simulink model "IceStorage_FHNW"  (R2018b)
settings: Solver=ode23  StartTime=-122*24*3600  StopTime=(365+181)*24*3600  EnableMultiTasking=on
StartFcn:
  | ticID_VsIceSTsim = tic;
StopFcn:
  | toc(ticID_VsIceSTsim)
undefined symbols (not defined in the file or in its folder): A, B, C, Davies, Dd, Hay
libraries: carnot x43, simulink x3, carsys x1
(part 2 of 2)

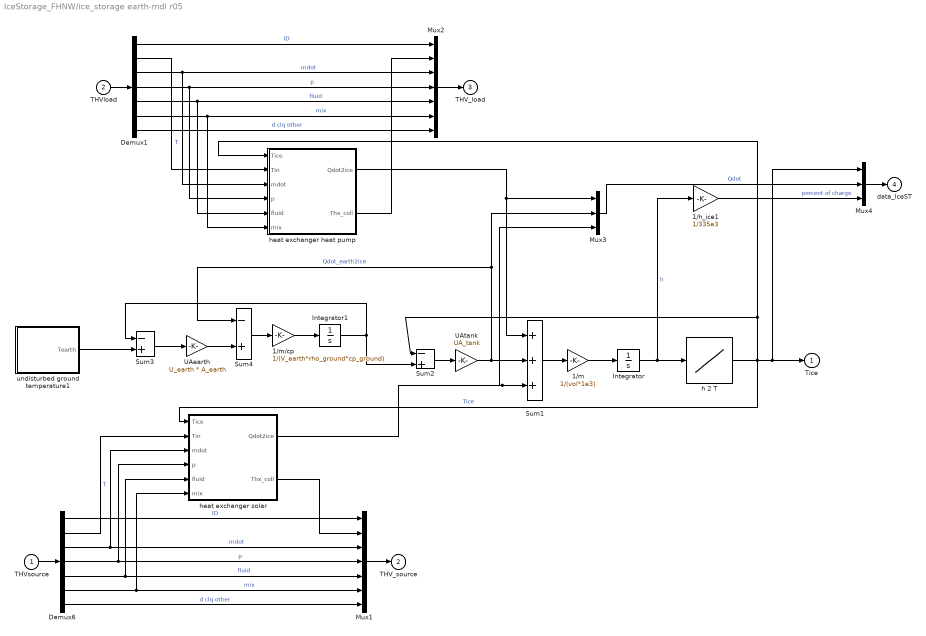
== system IceStorage_FHNW/ice_storage earth-mdl r05 ==
  THVsource : Inport
  THVload : Inport  Port=2
  1/h_ice1 : Gain  Gain=1/335e3  SaturateOnIntegerOverflow=on  OutDataTypeStr=Inherit: Same as input  ParamDataTypeStr=Inherit: Same as input
  1/m : Gain  Gain=1/(vol*1e3)  SaturateOnIntegerOverflow=on  OutDataTypeStr=Inherit: Same as input  ParamDataTypeStr=Inherit: Same as input
  1/m/cp : Gain  Gain=1/(V_earth*rho_ground*cp_ground)  SaturateOnIntegerOverflow=on  OutDataTypeStr=Inherit: Same as input  ParamDataTypeStr=Inherit: Same as input
  Demux1 : Demux  Outputs=[1 1 1 1 1 1 14]
  Demux6 : Demux  Outputs=[1 1 1 1 1 1 14]
  Integrator : Integrator  InitialCondition=h_ini
  Integrator1 : Integrator  InitialCondition=4
  Mux1 : Mux  Inputs=7
  Mux2 : Mux  Inputs=7
  Mux3 : Mux  Inputs=3
  Mux4 : Mux  Inputs=3
  Sum1 : Sum  Inputs=+++  SaturateOnIntegerOverflow=on  InputSameDT=on  OutDataTypeStr=Inherit: Same as first input
  Sum2 : Sum  Inputs=-+  SaturateOnIntegerOverflow=on  InputSameDT=on  OutDataTypeStr=Inherit: Same as first input
  Sum3 : Sum  Inputs=-+  SaturateOnIntegerOverflow=on  InputSameDT=on  OutDataTypeStr=Inherit: Same as first input
  Sum4 : Sum  Inputs=-+  SaturateOnIntegerOverflow=on  InputSameDT=on  OutDataTypeStr=Inherit: Same as first input
  UAearth : Gain  Gain=U_earth * A_earth  SaturateOnIntegerOverflow=on  OutDataTypeStr=Inherit: Same as input  ParamDataTypeStr=Inherit: Same as input
  UAtank : Gain  Gain=UA_tank  SaturateOnIntegerOverflow=on  OutDataTypeStr=Inherit: Same as input  ParamDataTypeStr=Inherit: Same as input
  h 2 T : Lookup  InputValues=[-2060*10 -2060*3 335e3 335e3+4182*10]  Table=[-10 -3 0 10]
  heat exchanger heat pump : Subsystem
  heat exchanger solar : Subsystem
  undisturbed ground temperature1 : Subsystem
  Tice : Outport  InitialOutput=0
  THV_source : Outport  Port=2  InitialOutput=0
  THV_load : Outport  Port=3  InitialOutput=0
  data_IceST : Outport  Port=4  InitialOutput=0
  wires:
  Mux3/1 -> Mux4/2  "Qdot"
  heat exchanger heat pump/1(Qdot2ice) -> Mux3/1, Sum1/1
  heat exchanger heat pump/2(Thx_coll) -> Mux2/2
  Demux1/2 -> heat exchanger heat pump/2(Tin)  "T"
  Demux1/6 -> Mux2/6, heat exchanger heat pump/6(mix)  "mix"
  Demux1/1 -> Mux2/1  "ID"
  Demux1/7 -> Mux2/7  "d clq other"
  Demux1/5 -> Mux2/5, heat exchanger heat pump/5(fluid)  "fluid"
  Demux1/4 -> Mux2/4, heat exchanger heat pump/4(p)  "p"
  Demux1/3 -> Mux2/3, heat exchanger heat pump/3(mdot)  "mdot"
  Mux2/1 -> THV_load/1
  THVload/1 -> Demux1/1
  heat exchanger solar/1(Qdot2ice) -> Mux3/3, Sum1/3
  h 2 T/1 -> Sum2/1, heat exchanger heat pump/1(Tice), heat exchanger solar/1(Tice), Mux4/1, Tice/1  "Tice"
  Integrator1/1 -> Sum3/1, Sum2/2
  1/m/cp/1 -> Integrator1/1
  Sum4/1 -> 1/m/cp/1
  UAearth/1 -> Sum4/2
  Sum3/1 -> UAearth/1
  Integrator/1 -> h 2 T/1, 1/h_ice1/1  "h"
  UAtank/1 -> Mux3/2, Sum4/1, Sum1/2  "Qdot_earth2ice"
  Sum2/1 -> UAtank/1
  Sum1/1 -> 1/m/1
  1/m/1 -> Integrator/1
  heat exchanger solar/2(Thx_coll) -> Mux1/2
  Demux6/2 -> heat exchanger solar/2(Tin)  "T"
  Demux6/6 -> heat exchanger solar/6(mix), Mux1/6  "mix"
  Demux6/1 -> Mux1/1  "ID"
  Demux6/7 -> Mux1/7  "d clq other"
  Demux6/5 -> heat exchanger solar/5(fluid), Mux1/5  "fluid"
  Demux6/4 -> heat exchanger solar/4(p), Mux1/4  "p"
  Demux6/3 -> heat exchanger solar/3(mdot), Mux1/3  "mdot"
  Mux1/1 -> THV_source/1
  THVsource/1 -> Demux6/1
  Mux4/1 -> data_IceST/1
  1/h_ice1/1 -> Mux4/3  "percent of charge"
  undisturbed ground temperature1/1(Tearth) -> Sum3/2

== system IceStorage_FHNW/measure_T ==
  THV_in : Inport
  heat capacity : StateSpace  A=-tc  B=tc  D=0  InitialCondition=t0
  select temperature : Selector  InputPortWidth=20  IndexOptions=Index vector (dialog)  Indices=[2]  OutputSizes=1
  T : Outport  InitialOutput=0
  wires:
  THV_in/1 -> select temperature/1
  select temperature/1 -> heat capacity/1
  heat capacity/1 -> T/1

== system IceStorage_FHNW/measure_T1 ==
  THV_in : Inport
  heat capacity : StateSpace  A=-tc  B=tc  D=0  InitialCondition=t0
  select temperature : Selector  InputPortWidth=20  IndexOptions=Index vector (dialog)  Indices=[2]  OutputSizes=1
  T : Outport  InitialOutput=0
  wires:
  heat capacity/1 -> T/1
  select temperature/1 -> heat capacity/1
  THV_in/1 -> select temperature/1

== system IceStorage_FHNW/measure_T2 ==
  THV_in : Inport
  heat capacity : StateSpace  A=-tc  B=tc  D=0  InitialCondition=t0
  select temperature : Selector  InputPortWidth=20  IndexOptions=Index vector (dialog)  Indices=[2]  OutputSizes=1
  T : Outport  InitialOutput=0
  wires:
  THV_in/1 -> select temperature/1
  select temperature/1 -> heat capacity/1
  heat capacity/1 -> T/1

== system IceStorage_FHNW/measure_T3 ==
  THV_in : Inport
  heat capacity : StateSpace  A=-tc  B=tc  D=0  InitialCondition=t0
  select temperature : Selector  InputPortWidth=20  IndexOptions=Index vector (dialog)  Indices=[2]  OutputSizes=1
  T : Outport  InitialOutput=0
  wires:
  THV_in/1 -> select temperature/1
  select temperature/1 -> heat capacity/1
  heat capacity/1 -> T/1

== system IceStorage_FHNW/measure_T4 ==
  THV_in : Inport
  heat capacity : StateSpace  A=-tc  B=tc  D=0  InitialCondition=t0
  select temperature : Selector  InputPortWidth=20  IndexOptions=Index vector (dialog)  Indices=[2]  OutputSizes=1
  T : Outport  InitialOutput=0
  wires:
  THV_in/1 -> select temperature/1
  select temperature/1 -> heat capacity/1
  heat capacity/1 -> T/1

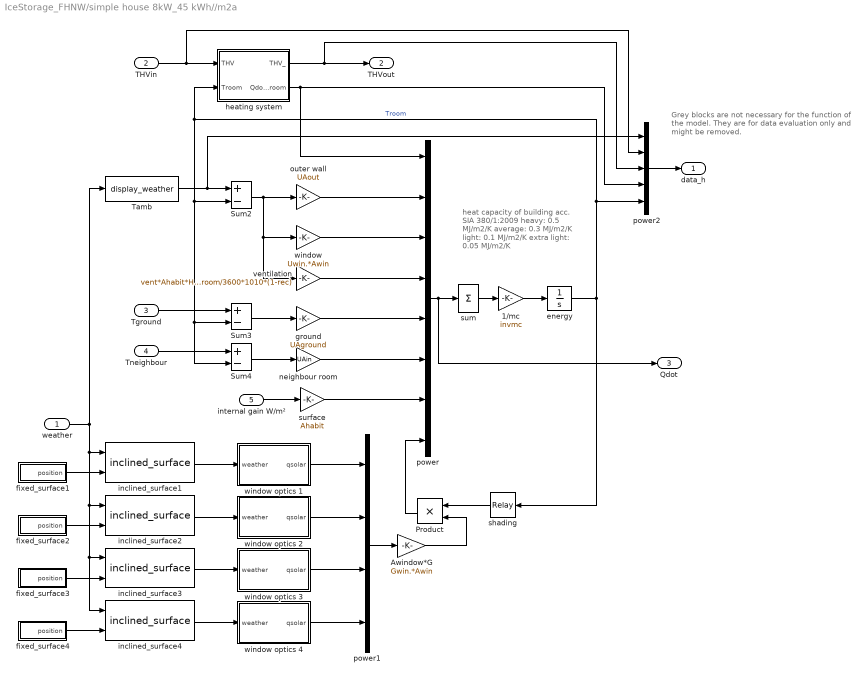
== system IceStorage_FHNW/simple house 8kW_45 kWh//m2a ==
  note: Grey blocks are not necessary for the function
      | of the model. They are for data evaluation only
      | and might be removed.
  note: heat capacity of building
      | acc. SIA 380/1:2009
      | heavy:          0.5 MJ/m2/K
      | average:       0.3 MJ/m2/K
      | light:            0.1 MJ/m2/K
      | extra light:  0.05 MJ/m2/K
  weather : Inport
  THVin : Inport  Port=2
  Tground : Inport  Port=3
  Tneighbour : Inport  Port=4
  internal gain W/m² : Inport  Port=5
  1/mc : Gain  Gain=invmc  SaturateOnIntegerOverflow=on  OutDataTypeStr=Inherit: Same as input  ParamDataTypeStr=Inherit: Same as input
  Awindow*G : Gain  Gain=Gwin.*Awin  SaturateOnIntegerOverflow=on  OutDataTypeStr=Inherit: Same as input  ParamDataTypeStr=Inherit: Same as input
  Product : Product  RndMeth=Zero
  Sum2 : Sum  Inputs=+-  SaturateOnIntegerOverflow=on  InputSameDT=on  OutDataTypeStr=Inherit: Same as first input
  Sum3 : Sum  Inputs=+-  SaturateOnIntegerOverflow=on  InputSameDT=on  OutDataTypeStr=Inherit: Same as first input
  Sum4 : Sum  Inputs=+-  SaturateOnIntegerOverflow=on  InputSameDT=on  OutDataTypeStr=Inherit: Same as first input
  Tamb : carnot/outputs/display_weather  pos=off  sun_dir=off  sun_dfu=off  rad=off  ta=on  ts=off  pre=off  rh=off  ci=off  p=off  ws=off  wd=off  col=off
      settings: SourceProductName=Carnot
  energy : Integrator  InitialCondition=tini
  fixed_surface1 : Subsystem  mask(fixed surface){colangle=90, colazi=AziWin(1), colrot=0}
      mask prompts: colangle "collector slope (0° = horizontal) [degree]"; colazi "collector azimuth (0° = south, -90° = east) [degree]"; colrot "collector rotation angle [degree]"
      mask help:
      | Set collector or surface to a fixed position.
      | All angles in degrees.
      mask init:
      | colangle = min(180, max(-180, colangle));
      | colazi = min(180, max(-180, colazi));
      | colrot = min(180, max(-180, colrot));
      mask Help: eval('htmlhelp (''chap_4_2f.htm#fixed_surface'')')
  fixed_surface2 : Subsystem  mask(fixed surface){colangle=90, colazi=AziWin(2), colrot=0}
      mask prompts: colangle "collector slope (0° = horizontal) [degree]"; colazi "collector azimuth (0° = south, -90° = east) [degree]"; colrot "collector rotation angle [degree]"
      mask help:
      | Set collector or surface to a fixed position.
      | All angles in degrees.
      mask init:
      | colangle = min(180, max(-180, colangle));
      | colazi = min(180, max(-180, colazi));
      | colrot = min(180, max(-180, colrot));
      mask Help: eval('htmlhelp (''chap_4_2f.htm#fixed_surface'')')
  fixed_surface3 : Subsystem  mask(fixed surface){colangle=90, colazi=AziWin(3), colrot=0}
      mask prompts: colangle "collector slope (0° = horizontal) [degree]"; colazi "collector azimuth (0° = south, -90° = east) [degree]"; colrot "collector rotation angle [degree]"
      mask help:
      | Set collector or surface to a fixed position.
      | All angles in degrees.
      mask init:
      | colangle = min(180, max(-180, colangle));
      | colazi = min(180, max(-180, colazi));
      | colrot = min(180, max(-180, colrot));
      mask Help: eval('htmlhelp (''chap_4_2f.htm#fixed_surface'')')
  fixed_surface4 : Subsystem  mask(fixed surface){colangle=90, colazi=AziWin(4), colrot=0}
      mask prompts: colangle "collector slope (0° = horizontal) [degree]"; colazi "collector azimuth (0° = south, -90° = east) [degree]"; colrot "collector rotation angle [degree]"
      mask help:
      | Set collector or surface to a fixed position.
      | All angles in degrees.
      mask init:
      | colangle = min(180, max(-180, colangle));
      | colazi = min(180, max(-180, colazi));
      | colrot = min(180, max(-180, colrot));
      mask Help: eval('htmlhelp (''chap_4_2f.htm#fixed_surface'')')
  ground : Gain  Gain=UAground  SaturateOnIntegerOverflow=on  OutDataTypeStr=Inherit: Same as input  ParamDataTypeStr=Inherit: Same as input
  heating system : Subsystem
  inclined_surface{1..4} (4 alike) : carnot/weather/inclined_surface  sky=Hay-Davies  reflect=0.2
      settings: SourceProductName=Carnot
  neighbour room : Gain  Gain=UAin  SaturateOnIntegerOverflow=on  OutDataTypeStr=Inherit: Same as input  ParamDataTypeStr=Inherit: Same as input
  outer wall : Gain  Gain=UAout  SaturateOnIntegerOverflow=on  OutDataTypeStr=Inherit: Same as input  ParamDataTypeStr=Inherit: Same as input
  power : Mux  Inputs=8
  power1 : Mux
  power2 : Mux  Inputs=5
  shading : Relay  OnSwitchValue=tini+4  OffSwitchValue=tini+3.5  OnOutputValue=1-shade  OffOutputValue=1
  sum : Sum  Inputs=1  SaturateOnIntegerOverflow=on  InputSameDT=on  OutDataTypeStr=Inherit: Same as first input
  surface : Gain  Gain=Ahabit  SaturateOnIntegerOverflow=on  OutDataTypeStr=Inherit: Same as input  ParamDataTypeStr=Inherit: Same as input
  ventilation : Gain  Gain=vent*Ahabit*Hroom/3600*1010*(1-rec)  SaturateOnIntegerOverflow=on  OutDataTypeStr=Inherit: Same as input  ParamDataTypeStr=Inherit: Same as input
  window : Gain  Gain=Uwin.*Awin  SaturateOnIntegerOverflow=on  OutDataTypeStr=Inherit: Same as input  ParamDataTypeStr=Inherit: Same as input
  window optics 1 : Subsystem
  window optics 2 : Subsystem
  window optics 3 : Subsystem
  window optics 4 : Subsystem
  data_h : Outport  InitialOutput=0
  THVout : Outport  Port=2  InitialOutput=0
  Qdot : Outport  Port=3  InitialOutput=0
  wires:
  1/mc/1 -> energy/1
  energy/1 -> Sum4/2, Sum3/2, Sum2/2, heating system/2(Troom), power2/5, shading/1  "Troom"
  sum/1 -> 1/mc/1
  inclined_surface4/1 -> window optics 4/1(weather)
  fixed_surface4/1(position) -> inclined_surface4/2
  inclined_surface3/1 -> window optics 3/1(weather)
  fixed_surface3/1(position) -> inclined_surface3/2
  inclined_surface2/1 -> window optics 2/1(weather)
  fixed_surface2/1(position) -> inclined_surface2/2
  power1/1 -> Awindow*G/1
  inclined_surface1/1 -> window optics 1/1(weather)
  fixed_surface1/1(position) -> inclined_surface1/2
  surface/1 -> power/7
  internal gain W/m²/1 -> surface/1
  neighbour room/1 -> power/6
  ground/1 -> power/5
  ventilation/1 -> power/4
  window/1 -> power/3
  Tneighbour/1 -> Sum4/1
  Sum4/1 -> neighbour room/1
  Tground/1 -> Sum3/1
  Sum3/1 -> ground/1
  heating system/1(THV_) -> THVout/1, power2/3
  THVin/1 -> heating system/1(THV), power2/2
  heating system/2(Qdot2room) -> power/1, power2/4
  power/1 -> sum/1, Qdot/1
  weather/1 -> inclined_surface4/1, inclined_surface3/1, inclined_surface2/1, inclined_surface1/1, Tamb/1
  Tamb/1 -> Sum2/1, power2/1
  outer wall/1 -> power/2
  Sum2/1 -> ventilation/1, window/1, outer wall/1
  power2/1 -> data_h/1
  shading/1 -> Product/1
  Awindow*G/1 -> Product/2
  Product/1 -> power/8
  window optics 1/1(qsolar) -> power1/1
  window optics 2/1(qsolar) -> power1/2
  window optics 3/1(qsolar) -> power1/3
  window optics 4/1(qsolar) -> power1/4

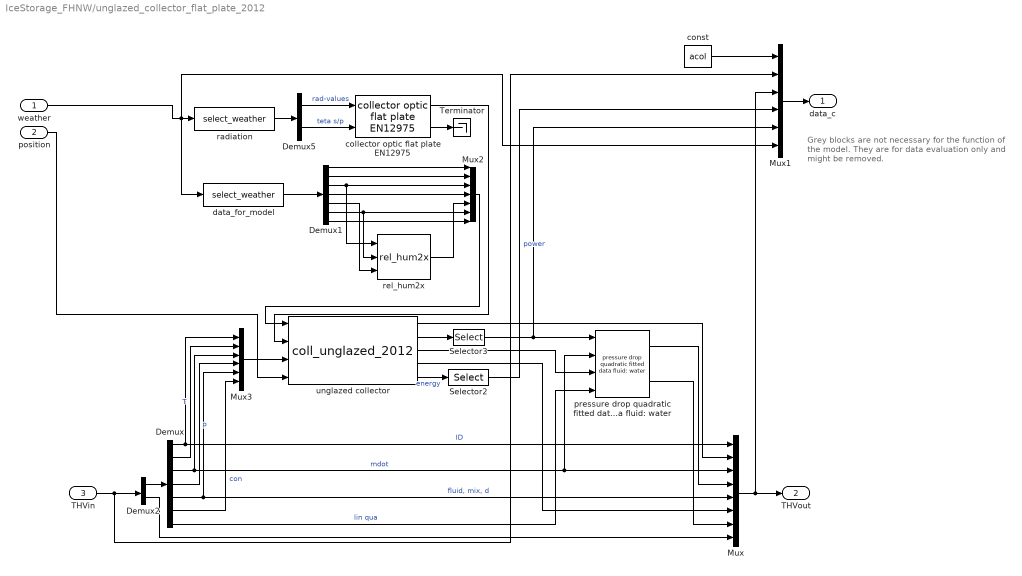
== system IceStorage_FHNW/unglazed_collector_flat_plate_2012 ==
  note: Grey blocks are not necessary for the function
      | of the model. They are for data evaluation only
      | and might be removed.
  weather : Inport
  position : Inport  Port=2
  THVin : Inport  Port=3
  Demux : Demux  Outputs=[1 1 1 1 3 1 2]
  Demux1 : Demux  Outputs=7
  Demux2 : Demux  Outputs=[10 10]
  Demux5 : Demux  Outputs=[5 2]
  Mux : Mux  Inputs=8
  Mux1 : Mux  Inputs=[1 20 20 1 1 -1]
  Mux2 : Mux  Inputs=7
  Mux3 : Mux  Inputs=6
  Selector2 : Selector  InputPortWidth=4  IndexOptions=Index vector (dialog)  Indices=[3]  OutputSizes=1
  Selector3 : Selector  InputPortWidth=6  IndexOptions=Index vector (dialog)  Indices=[6]  OutputSizes=1
  Terminator : Terminator
  collector optic flat plate EN12975 : carnot/heat_source/incidence angle modifier (IAM)/collector optic flat plate EN12975  b0=0  Kd=1
      settings: SourceProductName=Carnot
  const : Constant  Value=acol
  data_for_model : carnot/weather/select_weather  v=[16 17 5:7 10 11]  type_index=index of weather data vectors for CARNOT versions >= 5.1
      settings: SourceProductName=Carnot
  pressure drop quadratic fitted data fluid: water : carnot/heat_source/pressure drop of collector/pressure drop quadratic fitted data fluid: water  b=0.006201*3.6e5  a=0.000096*1.296e9  aonecol=2  acol=acol
      settings: SourceProductName=Carnot
  radiation : carnot/weather/select_weather  v=[1 2 13 16 17 14 15]  type_index=index of weather data vectors for CARNOT versions >= 5.1
      settings: SourceProductName=Carnot
  rel_hum2x : carnot/basics/rel_hum2x
      settings: SourceProductName=Carnot
  unglazed collector : S-Function  FunctionName=coll_unglazed_2012  Parameters=acol, uc0, uc1, uc0loss, uc1loss, uc0gain, uc1gain, e_sky, uc1eta0, hi, c_abs, c_fl, length, tini, nodes  SFunctionDeploymentMode=off  EnableBusSupport=off
  data_c : Outport  InitialOutput=0
  THVout : Outport  Port=2  InitialOutput=0
  wires:
  collector optic flat plate EN12975/1 -> unglazed collector/2
  Mux2/1 -> unglazed collector/1
  Demux1/4 -> Mux2/4
  rel_hum2x/1 -> Mux2/5
  Demux1/7 -> Mux2/7
  Demux1/2 -> Mux2/2
  Demux1/1 -> Mux2/1
  Demux1/5 -> rel_hum2x/3
  Demux1/6 -> Mux2/6, rel_hum2x/2
  Demux1/3 -> Mux2/3, rel_hum2x/1
  data_for_model/1 -> Demux1/1
  collector optic flat plate EN12975/2 -> Terminator/1
  unglazed collector/1 -> Mux/2
  unglazed collector/2 -> Selector3/1
  unglazed collector/3 -> pressure drop quadratic fitted data fluid: water/3
  unglazed collector/4 -> Mux/6
  Mux/1 -> THVout/1, Mux1/3
  Demux/3 -> Mux3/3, Mux/3, pressure drop quadratic fitted data fluid: water/2  "mdot"
  Demux/7 -> pressure drop quadratic fitted data fluid: water/4  "lin qua"
  Mux3/1 -> unglazed collector/3
  Demux5/2 -> collector optic flat plate EN12975/2  "teta s/p"
  Demux5/1 -> collector optic flat plate EN12975/1  "rad-values"
  radiation/1 -> Demux5/1
  position/1 -> unglazed collector/4
  weather/1 -> Mux1/6, radiation/1, data_for_model/1
  Demux/5 -> Mux/5, Mux3/5  "fluid, mix, d"
  Demux/1 -> Mux3/1, Mux/1  "ID"
  Demux2/1 -> Demux/1
  THVin/1 -> Demux2/1, Mux1/2
  Demux/4 -> Mux3/4  "p"
  Demux/2 -> Mux3/2  "T"
  Demux/6 -> Mux3/6  "con"
  pressure drop quadratic fitted data fluid: water/1 -> Mux/4
  Demux2/2 -> Mux/8
  pressure drop quadratic fitted data fluid: water/2 -> Mux/7
  unglazed collector/5 -> Selector2/1  "energy"
  Selector2/1 -> Mux1/4  "power"
  const/1 -> Mux1/1
  Mux1/1 -> data_c/1
  Selector3/1 -> pressure drop quadratic fitted data fluid: water/1, Mux1/5

== system IceStorage_FHNW/Viessmann_CVW_DHW_390_Liter/multiport storage ==
  Tamb : Inport
  port1 : Inport  Port=2
  port2 : Inport  Port=3
  port3 : Inport  Port=4
  S-Function : S-Function  FunctionName=generic_store  Parameters="d(1), d(2), 0, 0, pos, u(1), u(2), u(3), axialcond,  tinitial,  nodes, nport, 0, sensors"  SFunctionDeploymentMode=off  EnableBusSupport=off
  Tnodes : Outport  InitialOutput=0
  Energy : Outport  Port=2  InitialOutput=0
  "[T p]1" : Outport  Port=3  InitialOutput=0
  "[T p]2" : Outport  Port=4  InitialOutput=0
  "[T p]3" : Outport  Port=5  InitialOutput=0
  wires:
  S-Function/1 -> Tnodes/1
  port2/1 -> S-Function/3
  port1/1 -> S-Function/2
  Tamb/1 -> S-Function/1
  port3/1 -> S-Function/4
  S-Function/3 -> "[T p]1"/1
  S-Function/4 -> "[T p]2"/1
  S-Function/5 -> "[T p]3"/1
  S-Function/2 -> Energy/1

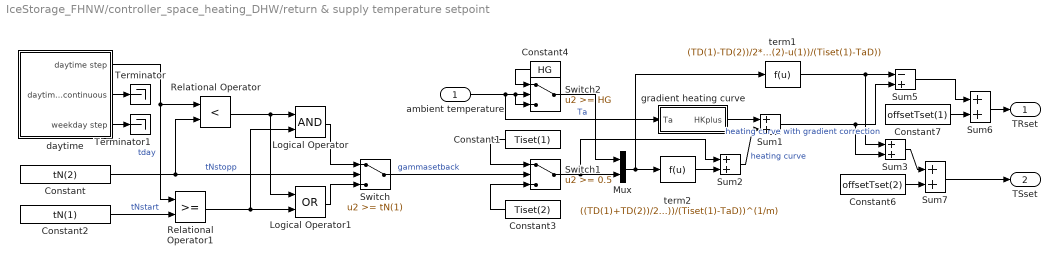
== system IceStorage_FHNW/controller_space_heating_DHW/return & supply temperature setpoint ==
  ambient temperature : Inport
  Constant : Constant  Value=tN(2)
  Constant1 : Constant  Value=Tiset(1)
  Constant2 : Constant  Value=tN(1)
  Constant3 : Constant  Value=Tiset(2)
  Constant4 : Constant  Value=HG
  Constant6 : Constant  Value=offsetTset(2)
  Constant7 : Constant  Value=offsetTset(1)
  Logical Operator : Logic
  Logical Operator1 : Logic  Operator=OR
  Mux : Mux  Inputs=2
  Relational Operator : RelationalOperator  Operator=<  RndMeth=Nearest  InputSameDT=on
  Relational Operator1 : RelationalOperator  RndMeth=Nearest  InputSameDT=on
  Sum{1..3,6..7} (5 alike) : Sum  SaturateOnIntegerOverflow=on  InputSameDT=on  OutDataTypeStr=Inherit: Same as first input
  Sum5 : Sum  Inputs=-+  SaturateOnIntegerOverflow=on  InputSameDT=on  OutDataTypeStr=Inherit: Same as first input
  Switch : Switch  Threshold=tN(1)  SaturateOnIntegerOverflow=on  InputSameDT=on
  Switch1 : Switch  Threshold=0.5  SaturateOnIntegerOverflow=on  InputSameDT=on
  Switch2 : Switch  Threshold=HG  SaturateOnIntegerOverflow=on  InputSameDT=on
  Terminator : Terminator
  Terminator1 : Terminator
  daytime : Subsystem
      mask help:
      | Evaluates the daytime and the weekday out of the simulation time.
      | The Decimation of the clock has to be adjusted under the mask in the clock parameter menu.
      | Output in seconds [s]
      mask Help:
      | created        10.2001  FHBB - IfE, suw
      | updated  22.01.2002  FHBB - IfE, suw / daytime continuous
      |                                                              / weekday step
      | 
      | The first weekday with simulation starttime zero is monday.
  gradient heating curve : Subsystem
  term1 : Fcn  Expr=(TD(1)-TD(2))/2*((u(2)-u(1))/(Tiset(1)-TaD))
  term2 : Fcn  Expr=((TD(1)+TD(2))/2-Tiset(1))*((u(2)-u(1))/(Tiset(1)-TaD))^(1/m)
  TRset : Outport
  TSset : Outport  Port=2
  wires:
  Switch2/1 -> Mux/1
  Constant4/1 -> Switch2/1
  Constant7/1 -> Sum6/2
  Constant6/1 -> Sum7/2
  Sum6/1 -> TRset/1
  Sum7/1 -> TSset/1
  term1/1 -> Sum5/1, Sum3/1
  Sum2/1 -> Sum1/2  "heating curve"
  Switch/1 -> Switch1/2  "gammasetback"
  Logical Operator1/1 -> Switch/3
  Switch1/1 -> Mux/2, Sum2/1
  Constant3/1 -> Switch1/3
  Constant1/1 -> Switch1/1
  Logical Operator/1 -> Switch/1
  Relational Operator1/1 -> Logical Operator1/2, Logical Operator/2
  Relational Operator/1 -> Logical Operator/1, Logical Operator1/1
  Constant2/1 -> Relational Operator1/2  "tNstart"
  Constant/1 -> Relational Operator/2, Switch/2  "tNstopp"
  daytime/1(daytime step) -> Relational Operator/1, Relational Operator1/1  "tday"
  ambient temperature/1 -> Switch2/2, Switch2/3, gradient heating curve/1(Ta)  "Ta"
  Mux/1 -> term2/1, term1/1
  term2/1 -> Sum2/2
  daytime/2(daytime continuous) -> Terminator/1
  daytime/3(weekday step) -> Terminator1/1
  Sum5/1 -> Sum6/1
  Sum3/1 -> Sum7/1
  Sum1/1 -> Sum5/2, Sum3/2  "heating curve with gradient correction"
  gradient heating curve/1(HKplus) -> Sum1/1

== system IceStorage_FHNW/controller_space_heating_DHW/schedule modi ==
  Clock : Clock
  Constant : Constant  Value=sim_start_time
  Fcn1 : Fcn  Expr=rem(u[1],period)
  Look-Up Table1 : Lookup  InputValues=rep_seq_t - min(rep_seq_t)  Table=rep_seq_y  SaturateOnIntegerOverflow=on
  Sum : Sum  Inputs=+-  SaturateOnIntegerOverflow=on  InputSameDT=on  OutDataTypeStr=Inherit: Same as first input
  Out1 : Outport
  wires:
  Fcn1/1 -> Look-Up Table1/1
  Look-Up Table1/1 -> Out1/1
  Sum/1 -> Fcn1/1
  Clock/1 -> Sum/1
  Constant/1 -> Sum/2

== system IceStorage_FHNW/controller_space_heating_DHW/value balance & hysteresis ==
  T : Inport
  Tset : Inport  Port=2
  Data Type Conversion3 : DataTypeConversion  OutDataTypeStr=double
  MinMax : MinMax  Function=max  Inputs=2  SaturateOnIntegerOverflow=on  InputSameDT=on
  Product : Product  SaturateOnIntegerOverflow=on  RndMeth=Zero  InputSameDT=on  OutDataTypeStr=Inherit: Same as first input
  Relational Operator2 : RelationalOperator  Operator=<=  RndMeth=Nearest  InputSameDT=on
  Relay : Relay  OnSwitchValue=deltaTRset(1)  OffSwitchValue=deltaTRset(2)
  Sum1 : Sum  Inputs=-+  SaturateOnIntegerOverflow=on  InputSameDT=on  OutDataTypeStr=Inherit: Same as first input
  Tmax option : Constant  Value=200
  signal : Outport
  wires:
  Data Type Conversion3/1 -> Product/2
  Sum1/1 -> Relay/1
  Tmax option/1 -> Relational Operator2/2
  MinMax/1 -> Relational Operator2/1
  Relay/1 -> Product/1  "gammaRset"
  Relational Operator2/1 -> Data Type Conversion3/1
  T/1 -> MinMax/1, Sum1/1  "T"
  Product/1 -> signal/1
  Tset/1 -> MinMax/2, Sum1/2  "Tset"

== system IceStorage_FHNW/controller_space_heating_DHW/value balance & hysteresis1 ==
  T : Inport
  Tset : Inport  Port=2
  Data Type Conversion3 : DataTypeConversion  OutDataTypeStr=double
  MinMax : MinMax  Function=max  Inputs=2  SaturateOnIntegerOverflow=on  InputSameDT=on
  Product : Product  SaturateOnIntegerOverflow=on  RndMeth=Zero  InputSameDT=on  OutDataTypeStr=Inherit: Same as first input
  Relational Operator2 : RelationalOperator  Operator=<=  RndMeth=Nearest  InputSameDT=on
  Relay : Relay  OnSwitchValue=deltaTRset(1)  OffSwitchValue=deltaTRset(2)
  Sum1 : Sum  Inputs=-+  SaturateOnIntegerOverflow=on  InputSameDT=on  OutDataTypeStr=Inherit: Same as first input
  Tmax option : Constant  Value=200
  signal : Outport
  wires:
  Data Type Conversion3/1 -> Product/2
  Tset/1 -> Sum1/2, MinMax/2  "Tset"
  Product/1 -> signal/1
  T/1 -> Sum1/1, MinMax/1  "T"
  Relational Operator2/1 -> Data Type Conversion3/1
  Relay/1 -> Product/1  "gammaRset"
  MinMax/1 -> Relational Operator2/1
  Tmax option/1 -> Relational Operator2/2
  Sum1/1 -> Relay/1

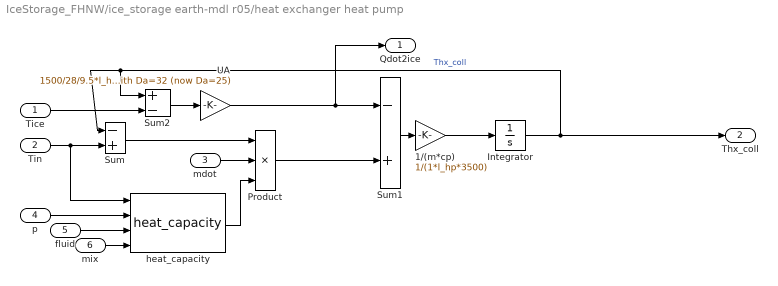
== system IceStorage_FHNW/ice_storage earth-mdl r05/heat exchanger heat pump ==
  Tice : Inport
  Tin : Inport  Port=2
  mdot : Inport  Port=3
  p : Inport  Port=4
  fluid : Inport  Port=5
  mix : Inport  Port=6
  1/(m*cp) : Gain  Gain=1/(1*l_hp*3500)  SaturateOnIntegerOverflow=on  OutDataTypeStr=Inherit: Same as input  ParamDataTypeStr=Inherit: Same as input
  Integrator : Integrator
  Product : Product  Inputs=3  SaturateOnIntegerOverflow=on  InputSameDT=on  OutDataTypeStr=Inherit: Same as first input
  Sum : Sum  Inputs=-+  SaturateOnIntegerOverflow=on  InputSameDT=on  OutDataTypeStr=Inherit: Same as first input
  Sum1 : Sum  Inputs=-+  SaturateOnIntegerOverflow=on  InputSameDT=on  OutDataTypeStr=Inherit: Same as first input
  Sum2 : Sum  Inputs=+-  SaturateOnIntegerOverflow=on  InputSameDT=on  OutDataTypeStr=Inherit: Same as first input
  UA : Gain  Gain="1500/28/9.5*l_hp*25/32            % 1.5 kW at 9 K on a 28 m tube with Da=32 (now Da=25)"  SaturateOnIntegerOverflow=on  OutDataTypeStr=Inherit: Same as input  ParamDataTypeStr=Inherit: Same as input
  heat_capacity : carnot/loads/simple house/heating system/radiator/heat_capacity
      settings: SourceProductName=Carnot
  Qdot2ice : Outport
  Thx_coll : Outport  Port=2
  wires:
  Tin/1 -> Sum/2, heat_capacity/1
  Integrator/1 -> Sum/1, Sum2/1, Thx_coll/1  "Thx_coll"
  Sum1/1 -> 1/(m*cp)/1
  Product/1 -> Sum1/2
  heat_capacity/1 -> Product/3
  Sum/1 -> Product/1
  Sum2/1 -> UA/1
  mdot/1 -> Product/2
  p/1 -> heat_capacity/2
  fluid/1 -> heat_capacity/3
  mix/1 -> heat_capacity/4
  Tice/1 -> Sum2/2
  1/(m*cp)/1 -> Integrator/1
  UA/1 -> Sum1/1, Qdot2ice/1

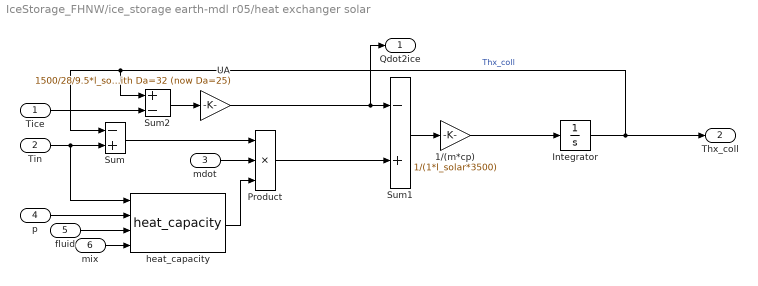
== system IceStorage_FHNW/ice_storage earth-mdl r05/heat exchanger solar ==
  Tice : Inport
  Tin : Inport  Port=2
  mdot : Inport  Port=3
  p : Inport  Port=4
  fluid : Inport  Port=5
  mix : Inport  Port=6
  1/(m*cp) : Gain  Gain=1/(1*l_solar*3500)  SaturateOnIntegerOverflow=on  OutDataTypeStr=Inherit: Same as input  ParamDataTypeStr=Inherit: Same as input
  Integrator : Integrator
  Product : Product  Inputs=3  SaturateOnIntegerOverflow=on  InputSameDT=on  OutDataTypeStr=Inherit: Same as first input
  Sum : Sum  Inputs=-+  SaturateOnIntegerOverflow=on  InputSameDT=on  OutDataTypeStr=Inherit: Same as first input
  Sum1 : Sum  Inputs=-+  SaturateOnIntegerOverflow=on  InputSameDT=on  OutDataTypeStr=Inherit: Same as first input
  Sum2 : Sum  Inputs=+-  SaturateOnIntegerOverflow=on  InputSameDT=on  OutDataTypeStr=Inherit: Same as first input
  UA : Gain  Gain="1500/28/9.5*l_solar*25/32            % 1.5 kW at 9 K on a 28 m tube with Da=32 (now Da=25)"  SaturateOnIntegerOverflow=on  OutDataTypeStr=Inherit: Same as input  ParamDataTypeStr=Inherit: Same as input
  heat_capacity : carnot/loads/simple house/heating system/radiator/heat_capacity
      settings: SourceProductName=Carnot
  Qdot2ice : Outport
  Thx_coll : Outport  Port=2
  wires:
  Tice/1 -> Sum2/2
  mix/1 -> heat_capacity/4
  fluid/1 -> heat_capacity/3
  p/1 -> heat_capacity/2
  mdot/1 -> Product/2
  Sum2/1 -> UA/1
  Sum/1 -> Product/1
  heat_capacity/1 -> Product/3
  Product/1 -> Sum1/2
  Sum1/1 -> 1/(m*cp)/1
  Integrator/1 -> Thx_coll/1, Sum2/1, Sum/1  "Thx_coll"
  Tin/1 -> heat_capacity/1, Sum/2
  1/(m*cp)/1 -> Integrator/1
  UA/1 -> Qdot2ice/1, Sum1/1

== system IceStorage_FHNW/ice_storage earth-mdl r05/undisturbed ground temperature1 ==
  Fcn : Fcn  Expr=u(1) - u(2)*exp(-u(3)/u(4))*cos(2*pi*(u(5)-u(6)*3600)/(365*24*3600) - u(3)/u(4)) + 0.03*u(3)
  Mux : Mux  Inputs=6
  Tmeanoutside : Constant  Value=Tmeanoutside
  delta_grd : Constant  Value=delta_grd
  deltathetae : Constant  Value=deltathetae
  depth of center of wall : Constant  Value=ztilde
  time : Clock
  tshift : Constant  Value=tshift
  Tearth : Outport
  wires:
  Fcn/1 -> Tearth/1
  Mux/1 -> Fcn/1
  tshift/1 -> Mux/6
  time/1 -> Mux/5
  delta_grd/1 -> Mux/4
  depth of center of wall/1 -> Mux/3
  deltathetae/1 -> Mux/2
  Tmeanoutside/1 -> Mux/1

== system IceStorage_FHNW/simple house 8kW_45 kWh//m2a/fixed_surface1 ==
  collector position : Constant  Value=[colangle colazi colrot]
  position : Outport  InitialOutput=0
  wires:
  collector position/1 -> position/1

== system IceStorage_FHNW/simple house 8kW_45 kWh//m2a/fixed_surface2 ==
  collector position : Constant  Value=[colangle colazi colrot]
  position : Outport  InitialOutput=0
  wires:
  collector position/1 -> position/1

== system IceStorage_FHNW/simple house 8kW_45 kWh//m2a/fixed_surface3 ==
  collector position : Constant  Value=[colangle colazi colrot]
  position : Outport  InitialOutput=0
  wires:
  collector position/1 -> position/1

== system IceStorage_FHNW/simple house 8kW_45 kWh//m2a/fixed_surface4 ==
  collector position : Constant  Value=[colangle colazi colrot]
  position : Outport  InitialOutput=0
  wires:
  collector position/1 -> position/1

== system IceStorage_FHNW/simple house 8kW_45 kWh//m2a/heating system ==
  THV : Inport
  Troom : Inport  Port=2
  Bias1 : Bias  Bias=dpcoeff
  Demux2 : Demux  Outputs=[1 1 1 1 1 1 1 1 2 10]
  Mux2 : Mux  Inputs=10
  pressuredrop_quadratic : carnot/basics/pressuredrop_quadratic  dplin=dpcoeff(1)  dpqua=dpcoeff(2)
      settings: SourceProductName=Carnot
  radiator : Subsystem
  THV_ : Outport
  Qdot2room : Outport  Port=2
  wires:
  Bias1/1 -> Mux2/9
  pressuredrop_quadratic/1 -> Mux2/4
  Mux2/1 -> THV_/1
  THV/1 -> Demux2/1
  radiator/2(Qdot) -> Qdot2room/1
  Troom/1 -> radiator/6(Troom)
  Demux2/6 -> radiator/4(mix), Mux2/6  "mix"
  Demux2/5 -> radiator/3(type), Mux2/5  "fluid"
  Demux2/4 -> pressuredrop_quadratic/2, radiator/2(p)  "p"
  Demux2/8 -> Mux2/8  "con"
  Demux2/10 -> Mux2/10
  Demux2/7 -> Mux2/7  "d"
  Demux2/1 -> Mux2/1  "ID"
  Demux2/9 -> Bias1/1  "lin_qua"
  Demux2/3 -> pressuredrop_quadratic/1, Mux2/3, radiator/1(mdot)  "mdot"
  Demux2/2 -> radiator/5(T)  "T"
  radiator/1(Tnode) -> Mux2/2

== system IceStorage_FHNW/simple house 8kW_45 kWh//m2a/window optics 1 ==
  weather : Inport
  Demux2 : Demux  Outputs=3
  Dot Product : DotProduct  InputSameDT=on  OutDataTypeStr=Inherit: Inherit via internal rule
  IAM diffuse : Gain  Gain=0.8  SaturateOnIntegerOverflow=on  OutDataTypeStr=Inherit: Same as input  ParamDataTypeStr=Inherit: Same as input
  IAM window : Lookup  InputValues=[0 50 70 80 90]  Table="[1.0  0.95  0.7  0.0  0.0]"  SaturateOnIntegerOverflow=on
  Sum : Sum  SaturateOnIntegerOverflow=on  InputSameDT=on  OutDataTypeStr=Inherit: Same as first input
  select_weather : carnot/weather/select_weather  v=[13 16 17]  type_index=index of weather data vectors for CARNOT versions >= 5.1
      settings: SourceProductName=Carnot
  qsolar : Outport  InitialOutput=0
  wires:
  Demux2/3 -> IAM diffuse/1  "Idir,tilt"
  IAM window/1 -> Dot Product/1
  IAM diffuse/1 -> Sum/2
  Dot Product/1 -> Sum/1
  Sum/1 -> qsolar/1
  Demux2/1 -> IAM window/1  "angle"
  Demux2/2 -> Dot Product/2  "Idir"
  weather/1 -> select_weather/1
  select_weather/1 -> Demux2/1

== system IceStorage_FHNW/simple house 8kW_45 kWh//m2a/window optics 2 ==
  weather : Inport
  Demux2 : Demux  Outputs=3
  Dot Product : DotProduct  InputSameDT=on  OutDataTypeStr=Inherit: Inherit via internal rule
  IAM diffuse : Gain  Gain=0.8  SaturateOnIntegerOverflow=on  OutDataTypeStr=Inherit: Same as input  ParamDataTypeStr=Inherit: Same as input
  IAM window : Lookup  InputValues=[0 50 70 80 90]  Table="[1.0  0.95  0.7  0.0  0.0]"  SaturateOnIntegerOverflow=on
  Sum : Sum  SaturateOnIntegerOverflow=on  InputSameDT=on  OutDataTypeStr=Inherit: Same as first input
  select_weather : carnot/weather/select_weather  v=[13 16 17]  type_index=index of weather data vectors for CARNOT versions >= 5.1
      settings: SourceProductName=Carnot
  qsolar : Outport  InitialOutput=0
  wires:
  select_weather/1 -> Demux2/1
  weather/1 -> select_weather/1
  Demux2/2 -> Dot Product/2  "Idir"
  Demux2/1 -> IAM window/1  "angle"
  Sum/1 -> qsolar/1
  Dot Product/1 -> Sum/1
  IAM diffuse/1 -> Sum/2
  IAM window/1 -> Dot Product/1
  Demux2/3 -> IAM diffuse/1  "Idir,tilt"

== system IceStorage_FHNW/simple house 8kW_45 kWh//m2a/window optics 3 ==
  weather : Inport
  Demux2 : Demux  Outputs=3
  Dot Product : DotProduct  InputSameDT=on  OutDataTypeStr=Inherit: Inherit via internal rule
  IAM diffuse : Gain  Gain=0.8  SaturateOnIntegerOverflow=on  OutDataTypeStr=Inherit: Same as input  ParamDataTypeStr=Inherit: Same as input
  IAM window : Lookup  InputValues=[0 50 70 80 90]  Table="[1.0  0.95  0.7  0.0  0.0]"  SaturateOnIntegerOverflow=on
  Sum : Sum  SaturateOnIntegerOverflow=on  InputSameDT=on  OutDataTypeStr=Inherit: Same as first input
  select_weather : carnot/weather/select_weather  v=[13 16 17]  type_index=index of weather data vectors for CARNOT versions >= 5.1
      settings: SourceProductName=Carnot
  qsolar : Outport  InitialOutput=0
  wires:
  Demux2/3 -> IAM diffuse/1  "Idir,tilt"
  IAM window/1 -> Dot Product/1
  IAM diffuse/1 -> Sum/2
  Dot Product/1 -> Sum/1
  Sum/1 -> qsolar/1
  Demux2/1 -> IAM window/1  "angle"
  Demux2/2 -> Dot Product/2  "Idir"
  weather/1 -> select_weather/1
  select_weather/1 -> Demux2/1

== system IceStorage_FHNW/simple house 8kW_45 kWh//m2a/window optics 4 ==
  weather : Inport
  Demux2 : Demux  Outputs=3
  Dot Product : DotProduct  InputSameDT=on  OutDataTypeStr=Inherit: Inherit via internal rule
  IAM diffuse : Gain  Gain=0.8  SaturateOnIntegerOverflow=on  OutDataTypeStr=Inherit: Same as input  ParamDataTypeStr=Inherit: Same as input
  IAM window : Lookup  InputValues=[0 50 70 80 90]  Table="[1.0  0.95  0.7  0.0  0.0]"  SaturateOnIntegerOverflow=on
  Sum : Sum  SaturateOnIntegerOverflow=on  InputSameDT=on  OutDataTypeStr=Inherit: Same as first input
  select_weather : carnot/weather/select_weather  v=[13 16 17]  type_index=index of weather data vectors for CARNOT versions >= 5.1
      settings: SourceProductName=Carnot
  qsolar : Outport  InitialOutput=0
  wires:
  select_weather/1 -> Demux2/1
  weather/1 -> select_weather/1
  Demux2/2 -> Dot Product/2  "Idir"
  Demux2/1 -> IAM window/1  "angle"
  Sum/1 -> qsolar/1
  Dot Product/1 -> Sum/1
  IAM diffuse/1 -> Sum/2
  IAM window/1 -> Dot Product/1
  Demux2/3 -> IAM diffuse/1  "Idir,tilt"

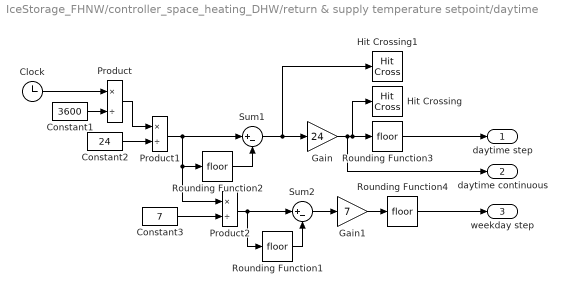
== system IceStorage_FHNW/controller_space_heating_DHW/return & supply temperature setpoint/daytime ==
  Clock : Clock
  Constant1 : Constant  Value=3600
  Constant2 : Constant  Value=24
  Constant3 : Constant  Value=7
  Gain : Gain  Gain=24  SaturateOnIntegerOverflow=on  OutDataTypeStr=Inherit: Same as input  ParamDataTypeStr=Inherit: Same as input
  Gain1 : Gain  Gain=7  SaturateOnIntegerOverflow=on  OutDataTypeStr=Inherit: Same as input  ParamDataTypeStr=Inherit: Same as input
  Hit Crossing : HitCross  HitCrossingOffset=[1 2 3 4 5 6 7 8 9 10 11 12 13 14 15 16 17 18 19 20 21 22 23]  ShowOutputPort=off
  Hit Crossing1 : HitCross  HitCrossingOffset=1  ShowOutputPort=off
  Product : Product  Inputs=*/  SaturateOnIntegerOverflow=on  RndMeth=Zero  InputSameDT=on  OutDataTypeStr=Inherit: Same as first input
  Product1 : Product  Inputs=*/  SaturateOnIntegerOverflow=on  RndMeth=Zero  InputSameDT=on  OutDataTypeStr=Inherit: Same as first input
  Product2 : Product  Inputs=*/  SaturateOnIntegerOverflow=on  RndMeth=Zero  InputSameDT=on  OutDataTypeStr=Inherit: Same as first input
  Rounding Function{1..4} (4 alike) : Rounding
  Sum1 : Sum  Inputs=|+-  SaturateOnIntegerOverflow=on  InputSameDT=on  OutDataTypeStr=Inherit: Same as first input
  Sum2 : Sum  Inputs=|+-  SaturateOnIntegerOverflow=on  InputSameDT=on  OutDataTypeStr=Inherit: Same as first input
  daytime step : Outport
  daytime continuous : Outport  Port=2
  weekday step : Outport  Port=3
  wires:
  Gain/1 -> Rounding Function3/1, Hit Crossing/1, daytime continuous/1
  Rounding Function3/1 -> daytime step/1
  Sum1/1 -> Hit Crossing1/1, Gain/1
  Rounding Function2/1 -> Sum1/2
  Product1/1 -> Sum1/1, Rounding Function2/1, Product2/1
  Constant2/1 -> Product1/2
  Product/1 -> Product1/1
  Constant1/1 -> Product/2
  Clock/1 -> Product/1
  Constant3/1 -> Product2/2
  Product2/1 -> Sum2/1, Rounding Function1/1
  Rounding Function1/1 -> Sum2/2
  Sum2/1 -> Gain1/1
  Gain1/1 -> Rounding Function4/1
  Rounding Function4/1 -> weekday step/1

== system IceStorage_FHNW/controller_space_heating_DHW/return & supply temperature setpoint/gradient heating curve ==
  Ta : Inport
  Constant : Constant  Value=deltaHK
  Constant1 : Constant  Value=Ta_deltaHK
  Constant2 : Constant  Value=TaD
  Product : Product  Inputs=*/*  SaturateOnIntegerOverflow=on  RndMeth=Zero  InputSameDT=on  OutDataTypeStr=Inherit: Same as first input
  Sum : Sum  Inputs=|+-  SaturateOnIntegerOverflow=on  InputSameDT=on  OutDataTypeStr=Inherit: Same as first input
  Sum1 : Sum  Inputs=-+|  SaturateOnIntegerOverflow=on  InputSameDT=on  OutDataTypeStr=Inherit: Same as first input
  HKplus : Outport
  wires:
  Constant/1 -> Product/1
  Constant1/1 -> Sum/1
  Sum/1 -> Product/2
  Constant2/1 -> Sum/2, Sum1/1
  Sum1/1 -> Product/3
  Product/1 -> HKplus/1
  Ta/1 -> Sum1/2

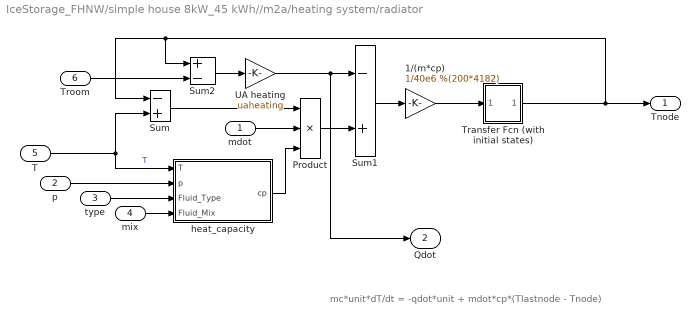
== system IceStorage_FHNW/simple house 8kW_45 kWh//m2a/heating system/radiator ==
  note: mc*unit*dT/dt = -qdot*unit + mdot*cp*(Tlastnode - Tnode)
  mdot : Inport
  p : Inport  Port=2
  type : Inport  Port=3
  mix : Inport  Port=4
  T : Inport  Port=5
  Troom : Inport  Port=6
  1/(m*cp) : Gain  Gain=1/40e6 %(200*4182)  SaturateOnIntegerOverflow=on  OutDataTypeStr=Inherit: Same as input  ParamDataTypeStr=Inherit: Same as input
  Product : Product  Inputs=3  SaturateOnIntegerOverflow=on  InputSameDT=on  OutDataTypeStr=Inherit: Same as first input
  Sum : Sum  Inputs=-+  SaturateOnIntegerOverflow=on  InputSameDT=on  OutDataTypeStr=Inherit: Same as first input
  Sum1 : Sum  Inputs=-+  SaturateOnIntegerOverflow=on  InputSameDT=on  OutDataTypeStr=Inherit: Same as first input
  Sum2 : Sum  Inputs=+-  SaturateOnIntegerOverflow=on  InputSameDT=on  OutDataTypeStr=Inherit: Same as first input
  Transfer Fcn (with initial states) : Subsystem  mask(Transfer Function with Initial States){N=[1], D=[1  0], X0=20}
      mask prompts: N "Numerator:"; D "Denominator:"; X0 "Initial conditions:"
      mask help: Vector expressions for numerator, and denominator. Coefficients are in descending powers of s.
      mask init:
      | [A,B,C,Dd]=tf2ss(N,D);if (isempty(X0));[m,n]=size(A);X0=zeros(1,m); end;
      mask Help: Specify the initial states for the transfer function.  The state ordering is determined by the m-file tf2ss.  There is no unique mapping of the states in a transfer function to states in a state-space representation.  However, tf2ss will consistently use the same mapping for a given transfer function.
      mask Display: dpoly(N,D,'s')
  UA heating : Gain  Gain=uaheating  SaturateOnIntegerOverflow=on  OutDataTypeStr=Inherit: Same as input  ParamDataTypeStr=Inherit: Same as input
  heat_capacity : Subsystem  mask(heat capacity){}
      mask help:
      | Calculates the  heat_capacity of fluids [J/(kg*K)].
      | Calls calls the function "hcap" in the CARNOT library "carlib".
      | Definition of the fluid types
      | fluid-ID  material           remarks on fluid mix
      | 1           water              vapourcontent in the 2-phase region
      | 2           air                   is (kg water) / (kg air)
      | 3           cotton oil
      | 4           silicone oil
      | 5           water-glycol    gives the volume partition [0..1] of glycol
      mask Help: eval('htmlhelp (''chap_4_2h.htm#heat_capacity'')')
  Tnode : Outport
  Qdot : Outport  Port=2
  wires:
  Transfer Fcn (with initial states)/1(Out1) -> Tnode/1, Sum/1, Sum2/1
  1/(m*cp)/1 -> Transfer Fcn (with initial states)/1(In1)
  Sum1/1 -> 1/(m*cp)/1
  Product/1 -> Sum1/2
  heat_capacity/1(cp) -> Product/3
  T/1 -> heat_capacity/1(T), Sum/2  "T"
  mdot/1 -> Product/2
  Sum/1 -> Product/1
  p/1 -> heat_capacity/2(p)
  type/1 -> heat_capacity/3(Fluid_Type)
  mix/1 -> heat_capacity/4(Fluid_Mix)
  Sum2/1 -> UA heating/1
  UA heating/1 -> Qdot/1, Sum1/1
  Troom/1 -> Sum2/2

== system IceStorage_FHNW/simple house 8kW_45 kWh//m2a/heating system/radiator/Transfer Fcn (with initial states) ==
  In1 : Inport
  State Space : StateSpace  A=A  B=B  C=C  D=Dd  InitialCondition=X0
  Out1 : Outport  InitialOutput=0
  wires:
  In1/1 -> State Space/1
  State Space/1 -> Out1/1

== system IceStorage_FHNW/simple house 8kW_45 kWh//m2a/heating system/radiator/heat_capacity ==
  T : Inport
  p : Inport  Port=2
  Fluid_Type : Inport  Port=3
  Fluid_Mix : Inport  Port=4
  S-Function : S-Function  FunctionName=capfluid  SFunctionDeploymentMode=off  EnableBusSupport=off
  cp : Outport  InitialOutput=0
  wires:
  p/1 -> S-Function/4
  T/1 -> S-Function/3
  Fluid_Mix/1 -> S-Function/2
  Fluid_Type/1 -> S-Function/1
  S-Function/1 -> cp/1
